simulink model "building_PHPP_v1"  (R2018b)
settings: Solver=ode23s  StartTime=-building.preruntime+8760*3600  StopTime=building.runtime+8760*3600  EnableMultiTasking=on
StartFcn:
  | tic
StopFcn:
  | toc
values from neighbouring files (symbols this model uses):
  A = 7*10*2    (= 140)    [theta_ground_v1.m]    (also in xlswrite1.m = num2cell(data))
  B = A/(0.5 * P)    (= 8.23529411765)    [theta_ground_v1.m]
  building = obj    [BUILDING.m]    (also in create_building_automatic.m = building.save(); ini_building_automatic.m = building.add_variant_hvac(building.variant_hvac, hvac); load_building_automatic.m = building.save())
  C = zeros(1,length(d)+1)    [CONSTRUCTION.m]    (also in DOOR.m = [0 0 0]; WALL.m = [0 0 0]; WINDOW.m = [0 0 0])
  cp = str2num(value)    [CONSTRUCTION.m]
  p = [timevec_weather weather(:,12)]    [BOUNDARY.m]    (also in WEATHER.m = 0; init_carnotUIBK.m = cell2mat(carnotUIBKpaths(i,2)))
  rho = str2num(value)    [CONSTRUCTION.m]    (also in theta_ground_v1.m = 2000)
undefined symbols (not defined in the file or in its folder): Dd, Dreifach, get_building, Qdot_C, Qdot_C_energy, Qdot_H, Qdot_H_energy, Qdot_I_electricity, Qdot_I_electricity_energy, Qdot_I_light, Qdot_I_light_energy, Qdot_I_person, Qdot_I_person_energy, Qdot_S, Qdot_S_energy, Qdot_T_ground, Qdot_T_ground_energy, Qdot_T_neighbour, Qdot_T_neighbour_energy, Qdot_T_opaque, Qdot_T_opaque_energy, Qdot_T_window, Qdot_T_window_energy, Qdot_V_infiltration, Qdot_V_infiltration_energy, Qdot_V_mech, Qdot_V_mech_energy, Qdot_V_window, Qdot_V_window_energy, Tc, Tr, Ts, Wärmeschutzglas, x_CO2, x_H2O, x_VOC
libraries: carnotUIBK x1874, carnot x5, simulink x3
(part 21 of 34)

== system building_PHPP_v1/BUILDING/INTERSECTION_5_8/wall_1 ==
  AIB1 : Inport
  AIB2 : Inport  Port=2
  Qdot_sol1 : Inport  Port=3
  Qdot_sol2 : Inport  Port=4
  EMPTY : carnotUIBK/wall_intersection/EMPTY  VariantControl=(default)
  R-C model : carnotUIBK/wall_intersection/R-C model  VariantControl=V_i_5_8_w1_m1  t0=z.t_ini  d=fliplr(const.parameter.xmesh_beu)  cond=fliplr(const.parameter.lambda)  cwall=fliplr(const.parameter.cp)  rho=fliplr(const.parameter.rho)  reflectground=0.2  abs_emiss=[const.absorption_2 const.emission_2 const.emission_1]  tau=const.parameter.tau  dactive=const.parameter.d_active
      link override alpha_i1/alpha_i_down: VariantControl=V_i_5_8_w1_hti2
      link override alpha_i1/alpha_i_horizontal: VariantControl=V_i_5_8_w1_hti0
      link override alpha_i1/alpha_i_up: VariantControl=V_i_5_8_w1_hti1
      link override alpha_i2/alpha_i_down: VariantControl=V_i_5_8_w1_hti2
      link override alpha_i2/alpha_i_horizontal: VariantControl=V_i_5_8_w1_hti0
      link override alpha_i2/alpha_i_up: VariantControl=V_i_5_8_w1_hti1
  UA : carnotUIBK/wall_intersection/UA  VariantControl=V_i_5_8_w1_m0  U=const.parameter.U
      link override Rsi/down: VariantControl=V_i_5_8_w1_hti2
      link override Rsi/horizontal: VariantControl=V_i_5_8_w1_hti0
      link override Rsi/up: VariantControl=V_i_5_8_w1_hti1
  hygrothermal model : carnotUIBK/wall_intersection/hygrothermal model  VariantControl=V_i_5_8_w1_m2  t0=z.t_ini  reflectground=0.2  abs_emiss=[const.absorption_2 const.emission_2 const.emission_1]  xmesh=const.parameter.xmesh_hygro  X=const.parameter.X  d=const.parameter.d  lambda=const.parameter.lambda_hygro  rho=const.parameter.rho_hygro  cp=const.parameter.cp_hygro  mu=const.parameter.mu  ufs=const.parameter.ufs  FSF_u=const.parameter.FSF_u  FSF_phi=const.parameter.FSF_phi  FSF_dudphi=const.parameter.FSF_dudphi  FSF_k=const.parameter.FSF_k  K_kleff=const.parameter.K_kleff  K_u=const.parameter.K_u  K_kl=const.parameter.K_kl  FSF_length=const.parameter.FSF_length  K_length=const.parameter.K_length  T_ini=const.parameter.T_ini_hygro  Phi_ini=const.parameter.Phi_ini_hygro  T_source=const.parameter.T_source  Phi_source=const.parameter.Phi_source  Tdactive=const.parameter.T_dactive  Phidactive=const.parameter.Phi_dactive
      link override alpha_i1/alpha_i_down: VariantControl=V_i_5_8_w1_hti2
      link override alpha_i1/alpha_i_horizontal: VariantControl=V_i_5_8_w1_hti0
      link override alpha_i1/alpha_i_up: VariantControl=V_i_5_8_w1_hti1
      link override alpha_i2/alpha_i_down: VariantControl=V_i_5_8_w1_hti2
      link override alpha_i2/alpha_i_horizontal: VariantControl=V_i_5_8_w1_hti0
      link override alpha_i2/alpha_i_up: VariantControl=V_i_5_8_w1_hti1
  "[S1]" : Outport
  "[S2]" : Outport  Port=2

== system building_PHPP_v1/BUILDING/INTERSECTION_5_8/wall_2 ==
  AIB1 : Inport
  AIB2 : Inport  Port=2
  Qdot_sol1 : Inport  Port=3
  Qdot_sol2 : Inport  Port=4
  EMPTY : carnotUIBK/wall_intersection/EMPTY  VariantControl=(default)
  R-C model : carnotUIBK/wall_intersection/R-C model  VariantControl=V_i_5_8_w2_m1  t0=z.t_ini  d=fliplr(const.parameter.xmesh_beu)  cond=fliplr(const.parameter.lambda)  cwall=fliplr(const.parameter.cp)  rho=fliplr(const.parameter.rho)  reflectground=0.2  abs_emiss=[const.absorption_2 const.emission_2 const.emission_1]  tau=const.parameter.tau  dactive=const.parameter.d_active
      link override alpha_i1/alpha_i_down: VariantControl=V_i_5_8_w2_hti2
      link override alpha_i1/alpha_i_horizontal: VariantControl=V_i_5_8_w2_hti0
      link override alpha_i1/alpha_i_up: VariantControl=V_i_5_8_w2_hti1
      link override alpha_i2/alpha_i_down: VariantControl=V_i_5_8_w2_hti2
      link override alpha_i2/alpha_i_horizontal: VariantControl=V_i_5_8_w2_hti0
      link override alpha_i2/alpha_i_up: VariantControl=V_i_5_8_w2_hti1
  UA : carnotUIBK/wall_intersection/UA  VariantControl=V_i_5_8_w2_m0  U=const.parameter.U
      link override Rsi/down: VariantControl=V_i_5_8_w2_hti2
      link override Rsi/horizontal: VariantControl=V_i_5_8_w2_hti0
      link override Rsi/up: VariantControl=V_i_5_8_w2_hti1
  hygrothermal model : carnotUIBK/wall_intersection/hygrothermal model  VariantControl=V_i_5_8_w2_m2  t0=z.t_ini  reflectground=0.2  abs_emiss=[const.absorption_2 const.emission_2 const.emission_1]  xmesh=const.parameter.xmesh_hygro  X=const.parameter.X  d=const.parameter.d  lambda=const.parameter.lambda_hygro  rho=const.parameter.rho_hygro  cp=const.parameter.cp_hygro  mu=const.parameter.mu  ufs=const.parameter.ufs  FSF_u=const.parameter.FSF_u  FSF_phi=const.parameter.FSF_phi  FSF_dudphi=const.parameter.FSF_dudphi  FSF_k=const.parameter.FSF_k  K_kleff=const.parameter.K_kleff  K_u=const.parameter.K_u  K_kl=const.parameter.K_kl  FSF_length=const.parameter.FSF_length  K_length=const.parameter.K_length  T_ini=const.parameter.T_ini_hygro  Phi_ini=const.parameter.Phi_ini_hygro  T_source=const.parameter.T_source  Phi_source=const.parameter.Phi_source  Tdactive=const.parameter.T_dactive  Phidactive=const.parameter.Phi_dactive
      link override alpha_i1/alpha_i_down: VariantControl=V_i_5_8_w2_hti2
      link override alpha_i1/alpha_i_horizontal: VariantControl=V_i_5_8_w2_hti0
      link override alpha_i1/alpha_i_up: VariantControl=V_i_5_8_w2_hti1
      link override alpha_i2/alpha_i_down: VariantControl=V_i_5_8_w2_hti2
      link override alpha_i2/alpha_i_horizontal: VariantControl=V_i_5_8_w2_hti0
      link override alpha_i2/alpha_i_up: VariantControl=V_i_5_8_w2_hti1
  "[S1]" : Outport
  "[S2]" : Outport  Port=2

== system building_PHPP_v1/BUILDING/INTERSECTION_5_8/wall_3 ==
  AIB1 : Inport
  AIB2 : Inport  Port=2
  Qdot_sol1 : Inport  Port=3
  Qdot_sol2 : Inport  Port=4
  EMPTY : carnotUIBK/wall_intersection/EMPTY  VariantControl=(default)
  R-C model : carnotUIBK/wall_intersection/R-C model  VariantControl=V_i_5_8_w3_m1  t0=z.t_ini  d=fliplr(const.parameter.xmesh_beu)  cond=fliplr(const.parameter.lambda)  cwall=fliplr(const.parameter.cp)  rho=fliplr(const.parameter.rho)  reflectground=0.2  abs_emiss=[const.absorption_2 const.emission_2 const.emission_1]  tau=const.parameter.tau  dactive=const.parameter.d_active
      link override alpha_i1/alpha_i_down: VariantControl=V_i_5_8_w3_hti2
      link override alpha_i1/alpha_i_horizontal: VariantControl=V_i_5_8_w3_hti0
      link override alpha_i1/alpha_i_up: VariantControl=V_i_5_8_w3_hti1
      link override alpha_i2/alpha_i_down: VariantControl=V_i_5_8_w3_hti2
      link override alpha_i2/alpha_i_horizontal: VariantControl=V_i_5_8_w3_hti0
      link override alpha_i2/alpha_i_up: VariantControl=V_i_5_8_w3_hti1
  UA : carnotUIBK/wall_intersection/UA  VariantControl=V_i_5_8_w3_m0  U=const.parameter.U
      link override Rsi/down: VariantControl=V_i_5_8_w3_hti2
      link override Rsi/horizontal: VariantControl=V_i_5_8_w3_hti0
      link override Rsi/up: VariantControl=V_i_5_8_w3_hti1
  hygrothermal model : carnotUIBK/wall_intersection/hygrothermal model  VariantControl=V_i_5_8_w3_m2  t0=z.t_ini  reflectground=0.2  abs_emiss=[const.absorption_2 const.emission_2 const.emission_1]  xmesh=const.parameter.xmesh_hygro  X=const.parameter.X  d=const.parameter.d  lambda=const.parameter.lambda_hygro  rho=const.parameter.rho_hygro  cp=const.parameter.cp_hygro  mu=const.parameter.mu  ufs=const.parameter.ufs  FSF_u=const.parameter.FSF_u  FSF_phi=const.parameter.FSF_phi  FSF_dudphi=const.parameter.FSF_dudphi  FSF_k=const.parameter.FSF_k  K_kleff=const.parameter.K_kleff  K_u=const.parameter.K_u  K_kl=const.parameter.K_kl  FSF_length=const.parameter.FSF_length  K_length=const.parameter.K_length  T_ini=const.parameter.T_ini_hygro  Phi_ini=const.parameter.Phi_ini_hygro  T_source=const.parameter.T_source  Phi_source=const.parameter.Phi_source  Tdactive=const.parameter.T_dactive  Phidactive=const.parameter.Phi_dactive
      link override alpha_i1/alpha_i_down: VariantControl=V_i_5_8_w3_hti2
      link override alpha_i1/alpha_i_horizontal: VariantControl=V_i_5_8_w3_hti0
      link override alpha_i1/alpha_i_up: VariantControl=V_i_5_8_w3_hti1
      link override alpha_i2/alpha_i_down: VariantControl=V_i_5_8_w3_hti2
      link override alpha_i2/alpha_i_horizontal: VariantControl=V_i_5_8_w3_hti0
      link override alpha_i2/alpha_i_up: VariantControl=V_i_5_8_w3_hti1
  "[S1]" : Outport
  "[S2]" : Outport  Port=2

== system building_PHPP_v1/BUILDING/INTERSECTION_5_9/airexchange_1 ==
  AIB1 : Inport
  AIB2 : Inport  Port=2
  control : Inport  Port=3
  EMPTY : carnotUIBK/airexchange_intersection/EMPTY  VariantControl=(default)
  airexchange_empiric : carnotUIBK/airexchange_intersection/airexchange_empiric  VariantControl=V_i_5_9_inf1_m0
  airexchange_powerlaw : carnotUIBK/airexchange_intersection/airexchange_powerlaw  VariantControl=V_i_5_9_inf1_m1
  "[S1]" : Outport
  "[S2]" : Outport  Port=2

== system building_PHPP_v1/BUILDING/INTERSECTION_5_9/airexchange_2 ==
  AIB1 : Inport
  AIB2 : Inport  Port=2
  control : Inport  Port=3
  EMPTY : carnotUIBK/airexchange_intersection/EMPTY  VariantControl=(default)
  airexchange_empiric : carnotUIBK/airexchange_intersection/airexchange_empiric  VariantControl=V_i_5_9_inf2_m0
  airexchange_powerlaw : carnotUIBK/airexchange_intersection/airexchange_powerlaw  VariantControl=V_i_5_9_inf2_m1
  "[S1]" : Outport
  "[S2]" : Outport  Port=2

== system building_PHPP_v1/BUILDING/INTERSECTION_5_9/airexchange_3 ==
  AIB1 : Inport
  AIB2 : Inport  Port=2
  control : Inport  Port=3
  EMPTY : carnotUIBK/airexchange_intersection/EMPTY  VariantControl=(default)
  airexchange_empiric : carnotUIBK/airexchange_intersection/airexchange_empiric  VariantControl=V_i_5_9_inf3_m0
  airexchange_powerlaw : carnotUIBK/airexchange_intersection/airexchange_powerlaw  VariantControl=V_i_5_9_inf3_m1
  "[S1]" : Outport
  "[S2]" : Outport  Port=2

== system building_PHPP_v1/BUILDING/INTERSECTION_5_9/wall_1 ==
  AIB1 : Inport
  AIB2 : Inport  Port=2
  Qdot_sol1 : Inport  Port=3
  Qdot_sol2 : Inport  Port=4
  EMPTY : carnotUIBK/wall_intersection/EMPTY  VariantControl=(default)
  R-C model : carnotUIBK/wall_intersection/R-C model  VariantControl=V_i_5_9_w1_m1  t0=z.t_ini  d=fliplr(const.parameter.xmesh_beu)  cond=fliplr(const.parameter.lambda)  cwall=fliplr(const.parameter.cp)  rho=fliplr(const.parameter.rho)  reflectground=0.2  abs_emiss=[const.absorption_2 const.emission_2 const.emission_1]  tau=const.parameter.tau  dactive=const.parameter.d_active
      link override alpha_i1/alpha_i_down: VariantControl=V_i_5_9_w1_hti2
      link override alpha_i1/alpha_i_horizontal: VariantControl=V_i_5_9_w1_hti0
      link override alpha_i1/alpha_i_up: VariantControl=V_i_5_9_w1_hti1
      link override alpha_i2/alpha_i_down: VariantControl=V_i_5_9_w1_hti2
      link override alpha_i2/alpha_i_horizontal: VariantControl=V_i_5_9_w1_hti0
      link override alpha_i2/alpha_i_up: VariantControl=V_i_5_9_w1_hti1
  UA : carnotUIBK/wall_intersection/UA  VariantControl=V_i_5_9_w1_m0  U=const.parameter.U
      link override Rsi/down: VariantControl=V_i_5_9_w1_hti2
      link override Rsi/horizontal: VariantControl=V_i_5_9_w1_hti0
      link override Rsi/up: VariantControl=V_i_5_9_w1_hti1
  hygrothermal model : carnotUIBK/wall_intersection/hygrothermal model  VariantControl=V_i_5_9_w1_m2  t0=z.t_ini  reflectground=0.2  abs_emiss=[const.absorption_2 const.emission_2 const.emission_1]  xmesh=const.parameter.xmesh_hygro  X=const.parameter.X  d=const.parameter.d  lambda=const.parameter.lambda_hygro  rho=const.parameter.rho_hygro  cp=const.parameter.cp_hygro  mu=const.parameter.mu  ufs=const.parameter.ufs  FSF_u=const.parameter.FSF_u  FSF_phi=const.parameter.FSF_phi  FSF_dudphi=const.parameter.FSF_dudphi  FSF_k=const.parameter.FSF_k  K_kleff=const.parameter.K_kleff  K_u=const.parameter.K_u  K_kl=const.parameter.K_kl  FSF_length=const.parameter.FSF_length  K_length=const.parameter.K_length  T_ini=const.parameter.T_ini_hygro  Phi_ini=const.parameter.Phi_ini_hygro  T_source=const.parameter.T_source  Phi_source=const.parameter.Phi_source  Tdactive=const.parameter.T_dactive  Phidactive=const.parameter.Phi_dactive
      link override alpha_i1/alpha_i_down: VariantControl=V_i_5_9_w1_hti2
      link override alpha_i1/alpha_i_horizontal: VariantControl=V_i_5_9_w1_hti0
      link override alpha_i1/alpha_i_up: VariantControl=V_i_5_9_w1_hti1
      link override alpha_i2/alpha_i_down: VariantControl=V_i_5_9_w1_hti2
      link override alpha_i2/alpha_i_horizontal: VariantControl=V_i_5_9_w1_hti0
      link override alpha_i2/alpha_i_up: VariantControl=V_i_5_9_w1_hti1
  "[S1]" : Outport
  "[S2]" : Outport  Port=2

== system building_PHPP_v1/BUILDING/INTERSECTION_5_9/wall_2 ==
  AIB1 : Inport
  AIB2 : Inport  Port=2
  Qdot_sol1 : Inport  Port=3
  Qdot_sol2 : Inport  Port=4
  EMPTY : carnotUIBK/wall_intersection/EMPTY  VariantControl=(default)
  R-C model : carnotUIBK/wall_intersection/R-C model  VariantControl=V_i_5_9_w2_m1  t0=z.t_ini  d=fliplr(const.parameter.xmesh_beu)  cond=fliplr(const.parameter.lambda)  cwall=fliplr(const.parameter.cp)  rho=fliplr(const.parameter.rho)  reflectground=0.2  abs_emiss=[const.absorption_2 const.emission_2 const.emission_1]  tau=const.parameter.tau  dactive=const.parameter.d_active
      link override alpha_i1/alpha_i_down: VariantControl=V_i_5_9_w2_hti2
      link override alpha_i1/alpha_i_horizontal: VariantControl=V_i_5_9_w2_hti0
      link override alpha_i1/alpha_i_up: VariantControl=V_i_5_9_w2_hti1
      link override alpha_i2/alpha_i_down: VariantControl=V_i_5_9_w2_hti2
      link override alpha_i2/alpha_i_horizontal: VariantControl=V_i_5_9_w2_hti0
      link override alpha_i2/alpha_i_up: VariantControl=V_i_5_9_w2_hti1
  UA : carnotUIBK/wall_intersection/UA  VariantControl=V_i_5_9_w2_m0  U=const.parameter.U
      link override Rsi/down: VariantControl=V_i_5_9_w2_hti2
      link override Rsi/horizontal: VariantControl=V_i_5_9_w2_hti0
      link override Rsi/up: VariantControl=V_i_5_9_w2_hti1
  hygrothermal model : carnotUIBK/wall_intersection/hygrothermal model  VariantControl=V_i_5_9_w2_m2  t0=z.t_ini  reflectground=0.2  abs_emiss=[const.absorption_2 const.emission_2 const.emission_1]  xmesh=const.parameter.xmesh_hygro  X=const.parameter.X  d=const.parameter.d  lambda=const.parameter.lambda_hygro  rho=const.parameter.rho_hygro  cp=const.parameter.cp_hygro  mu=const.parameter.mu  ufs=const.parameter.ufs  FSF_u=const.parameter.FSF_u  FSF_phi=const.parameter.FSF_phi  FSF_dudphi=const.parameter.FSF_dudphi  FSF_k=const.parameter.FSF_k  K_kleff=const.parameter.K_kleff  K_u=const.parameter.K_u  K_kl=const.parameter.K_kl  FSF_length=const.parameter.FSF_length  K_length=const.parameter.K_length  T_ini=const.parameter.T_ini_hygro  Phi_ini=const.parameter.Phi_ini_hygro  T_source=const.parameter.T_source  Phi_source=const.parameter.Phi_source  Tdactive=const.parameter.T_dactive  Phidactive=const.parameter.Phi_dactive
      link override alpha_i1/alpha_i_down: VariantControl=V_i_5_9_w2_hti2
      link override alpha_i1/alpha_i_horizontal: VariantControl=V_i_5_9_w2_hti0
      link override alpha_i1/alpha_i_up: VariantControl=V_i_5_9_w2_hti1
      link override alpha_i2/alpha_i_down: VariantControl=V_i_5_9_w2_hti2
      link override alpha_i2/alpha_i_horizontal: VariantControl=V_i_5_9_w2_hti0
      link override alpha_i2/alpha_i_up: VariantControl=V_i_5_9_w2_hti1
  "[S1]" : Outport
  "[S2]" : Outport  Port=2

== system building_PHPP_v1/BUILDING/INTERSECTION_5_9/wall_3 ==
  AIB1 : Inport
  AIB2 : Inport  Port=2
  Qdot_sol1 : Inport  Port=3
  Qdot_sol2 : Inport  Port=4
  EMPTY : carnotUIBK/wall_intersection/EMPTY  VariantControl=(default)
  R-C model : carnotUIBK/wall_intersection/R-C model  VariantControl=V_i_5_9_w3_m1  t0=z.t_ini  d=fliplr(const.parameter.xmesh_beu)  cond=fliplr(const.parameter.lambda)  cwall=fliplr(const.parameter.cp)  rho=fliplr(const.parameter.rho)  reflectground=0.2  abs_emiss=[const.absorption_2 const.emission_2 const.emission_1]  tau=const.parameter.tau  dactive=const.parameter.d_active
      link override alpha_i1/alpha_i_down: VariantControl=V_i_5_9_w3_hti2
      link override alpha_i1/alpha_i_horizontal: VariantControl=V_i_5_9_w3_hti0
      link override alpha_i1/alpha_i_up: VariantControl=V_i_5_9_w3_hti1
      link override alpha_i2/alpha_i_down: VariantControl=V_i_5_9_w3_hti2
      link override alpha_i2/alpha_i_horizontal: VariantControl=V_i_5_9_w3_hti0
      link override alpha_i2/alpha_i_up: VariantControl=V_i_5_9_w3_hti1
  UA : carnotUIBK/wall_intersection/UA  VariantControl=V_i_5_9_w3_m0  U=const.parameter.U
      link override Rsi/down: VariantControl=V_i_5_9_w3_hti2
      link override Rsi/horizontal: VariantControl=V_i_5_9_w3_hti0
      link override Rsi/up: VariantControl=V_i_5_9_w3_hti1
  hygrothermal model : carnotUIBK/wall_intersection/hygrothermal model  VariantControl=V_i_5_9_w3_m2  t0=z.t_ini  reflectground=0.2  abs_emiss=[const.absorption_2 const.emission_2 const.emission_1]  xmesh=const.parameter.xmesh_hygro  X=const.parameter.X  d=const.parameter.d  lambda=const.parameter.lambda_hygro  rho=const.parameter.rho_hygro  cp=const.parameter.cp_hygro  mu=const.parameter.mu  ufs=const.parameter.ufs  FSF_u=const.parameter.FSF_u  FSF_phi=const.parameter.FSF_phi  FSF_dudphi=const.parameter.FSF_dudphi  FSF_k=const.parameter.FSF_k  K_kleff=const.parameter.K_kleff  K_u=const.parameter.K_u  K_kl=const.parameter.K_kl  FSF_length=const.parameter.FSF_length  K_length=const.parameter.K_length  T_ini=const.parameter.T_ini_hygro  Phi_ini=const.parameter.Phi_ini_hygro  T_source=const.parameter.T_source  Phi_source=const.parameter.Phi_source  Tdactive=const.parameter.T_dactive  Phidactive=const.parameter.Phi_dactive
      link override alpha_i1/alpha_i_down: VariantControl=V_i_5_9_w3_hti2
      link override alpha_i1/alpha_i_horizontal: VariantControl=V_i_5_9_w3_hti0
      link override alpha_i1/alpha_i_up: VariantControl=V_i_5_9_w3_hti1
      link override alpha_i2/alpha_i_down: VariantControl=V_i_5_9_w3_hti2
      link override alpha_i2/alpha_i_horizontal: VariantControl=V_i_5_9_w3_hti0
      link override alpha_i2/alpha_i_up: VariantControl=V_i_5_9_w3_hti1
  "[S1]" : Outport
  "[S2]" : Outport  Port=2

== system building_PHPP_v1/BUILDING/INTERSECTION_6_10/airexchange_1 ==
  AIB1 : Inport
  AIB2 : Inport  Port=2
  control : Inport  Port=3
  EMPTY : carnotUIBK/airexchange_intersection/EMPTY  VariantControl=(default)
  airexchange_empiric : carnotUIBK/airexchange_intersection/airexchange_empiric  VariantControl=V_i_6_10_inf1_m0
  airexchange_powerlaw : carnotUIBK/airexchange_intersection/airexchange_powerlaw  VariantControl=V_i_6_10_inf1_m1
  "[S1]" : Outport
  "[S2]" : Outport  Port=2

== system building_PHPP_v1/BUILDING/INTERSECTION_6_10/airexchange_2 ==
  AIB1 : Inport
  AIB2 : Inport  Port=2
  control : Inport  Port=3
  EMPTY : carnotUIBK/airexchange_intersection/EMPTY  VariantControl=(default)
  airexchange_empiric : carnotUIBK/airexchange_intersection/airexchange_empiric  VariantControl=V_i_6_10_inf2_m0
  airexchange_powerlaw : carnotUIBK/airexchange_intersection/airexchange_powerlaw  VariantControl=V_i_6_10_inf2_m1
  "[S1]" : Outport
  "[S2]" : Outport  Port=2

== system building_PHPP_v1/BUILDING/INTERSECTION_6_10/airexchange_3 ==
  AIB1 : Inport
  AIB2 : Inport  Port=2
  control : Inport  Port=3
  EMPTY : carnotUIBK/airexchange_intersection/EMPTY  VariantControl=(default)
  airexchange_empiric : carnotUIBK/airexchange_intersection/airexchange_empiric  VariantControl=V_i_6_10_inf3_m0
  airexchange_powerlaw : carnotUIBK/airexchange_intersection/airexchange_powerlaw  VariantControl=V_i_6_10_inf3_m1
  "[S1]" : Outport
  "[S2]" : Outport  Port=2

== system building_PHPP_v1/BUILDING/INTERSECTION_6_10/wall_1 ==
  AIB1 : Inport
  AIB2 : Inport  Port=2
  Qdot_sol1 : Inport  Port=3
  Qdot_sol2 : Inport  Port=4
  EMPTY : carnotUIBK/wall_intersection/EMPTY  VariantControl=(default)
  R-C model : carnotUIBK/wall_intersection/R-C model  VariantControl=V_i_6_10_w1_m1  t0=z.t_ini  d=fliplr(const.parameter.xmesh_beu)  cond=fliplr(const.parameter.lambda)  cwall=fliplr(const.parameter.cp)  rho=fliplr(const.parameter.rho)  reflectground=0.2  abs_emiss=[const.absorption_2 const.emission_2 const.emission_1]  tau=const.parameter.tau  dactive=const.parameter.d_active
      link override alpha_i1/alpha_i_down: VariantControl=V_i_6_10_w1_hti2
      link override alpha_i1/alpha_i_horizontal: VariantControl=V_i_6_10_w1_hti0
      link override alpha_i1/alpha_i_up: VariantControl=V_i_6_10_w1_hti1
      link override alpha_i2/alpha_i_down: VariantControl=V_i_6_10_w1_hti2
      link override alpha_i2/alpha_i_horizontal: VariantControl=V_i_6_10_w1_hti0
      link override alpha_i2/alpha_i_up: VariantControl=V_i_6_10_w1_hti1
  UA : carnotUIBK/wall_intersection/UA  VariantControl=V_i_6_10_w1_m0  U=const.parameter.U
      link override Rsi/down: VariantControl=V_i_6_10_w1_hti2
      link override Rsi/horizontal: VariantControl=V_i_6_10_w1_hti0
      link override Rsi/up: VariantControl=V_i_6_10_w1_hti1
  hygrothermal model : carnotUIBK/wall_intersection/hygrothermal model  VariantControl=V_i_6_10_w1_m2  t0=z.t_ini  reflectground=0.2  abs_emiss=[const.absorption_2 const.emission_2 const.emission_1]  xmesh=const.parameter.xmesh_hygro  X=const.parameter.X  d=const.parameter.d  lambda=const.parameter.lambda_hygro  rho=const.parameter.rho_hygro  cp=const.parameter.cp_hygro  mu=const.parameter.mu  ufs=const.parameter.ufs  FSF_u=const.parameter.FSF_u  FSF_phi=const.parameter.FSF_phi  FSF_dudphi=const.parameter.FSF_dudphi  FSF_k=const.parameter.FSF_k  K_kleff=const.parameter.K_kleff  K_u=const.parameter.K_u  K_kl=const.parameter.K_kl  FSF_length=const.parameter.FSF_length  K_length=const.parameter.K_length  T_ini=const.parameter.T_ini_hygro  Phi_ini=const.parameter.Phi_ini_hygro  T_source=const.parameter.T_source  Phi_source=const.parameter.Phi_source  Tdactive=const.parameter.T_dactive  Phidactive=const.parameter.Phi_dactive
      link override alpha_i1/alpha_i_down: VariantControl=V_i_6_10_w1_hti2
      link override alpha_i1/alpha_i_horizontal: VariantControl=V_i_6_10_w1_hti0
      link override alpha_i1/alpha_i_up: VariantControl=V_i_6_10_w1_hti1
      link override alpha_i2/alpha_i_down: VariantControl=V_i_6_10_w1_hti2
      link override alpha_i2/alpha_i_horizontal: VariantControl=V_i_6_10_w1_hti0
      link override alpha_i2/alpha_i_up: VariantControl=V_i_6_10_w1_hti1
  "[S1]" : Outport
  "[S2]" : Outport  Port=2

== system building_PHPP_v1/BUILDING/INTERSECTION_6_10/wall_2 ==
  AIB1 : Inport
  AIB2 : Inport  Port=2
  Qdot_sol1 : Inport  Port=3
  Qdot_sol2 : Inport  Port=4
  EMPTY : carnotUIBK/wall_intersection/EMPTY  VariantControl=(default)
  R-C model : carnotUIBK/wall_intersection/R-C model  VariantControl=V_i_6_10_w2_m1  t0=z.t_ini  d=fliplr(const.parameter.xmesh_beu)  cond=fliplr(const.parameter.lambda)  cwall=fliplr(const.parameter.cp)  rho=fliplr(const.parameter.rho)  reflectground=0.2  abs_emiss=[const.absorption_2 const.emission_2 const.emission_1]  tau=const.parameter.tau  dactive=const.parameter.d_active
      link override alpha_i1/alpha_i_down: VariantControl=V_i_6_10_w2_hti2
      link override alpha_i1/alpha_i_horizontal: VariantControl=V_i_6_10_w2_hti0
      link override alpha_i1/alpha_i_up: VariantControl=V_i_6_10_w2_hti1
      link override alpha_i2/alpha_i_down: VariantControl=V_i_6_10_w2_hti2
      link override alpha_i2/alpha_i_horizontal: VariantControl=V_i_6_10_w2_hti0
      link override alpha_i2/alpha_i_up: VariantControl=V_i_6_10_w2_hti1
  UA : carnotUIBK/wall_intersection/UA  VariantControl=V_i_6_10_w2_m0  U=const.parameter.U
      link override Rsi/down: VariantControl=V_i_6_10_w2_hti2
      link override Rsi/horizontal: VariantControl=V_i_6_10_w2_hti0
      link override Rsi/up: VariantControl=V_i_6_10_w2_hti1
  hygrothermal model : carnotUIBK/wall_intersection/hygrothermal model  VariantControl=V_i_6_10_w2_m2  t0=z.t_ini  reflectground=0.2  abs_emiss=[const.absorption_2 const.emission_2 const.emission_1]  xmesh=const.parameter.xmesh_hygro  X=const.parameter.X  d=const.parameter.d  lambda=const.parameter.lambda_hygro  rho=const.parameter.rho_hygro  cp=const.parameter.cp_hygro  mu=const.parameter.mu  ufs=const.parameter.ufs  FSF_u=const.parameter.FSF_u  FSF_phi=const.parameter.FSF_phi  FSF_dudphi=const.parameter.FSF_dudphi  FSF_k=const.parameter.FSF_k  K_kleff=const.parameter.K_kleff  K_u=const.parameter.K_u  K_kl=const.parameter.K_kl  FSF_length=const.parameter.FSF_length  K_length=const.parameter.K_length  T_ini=const.parameter.T_ini_hygro  Phi_ini=const.parameter.Phi_ini_hygro  T_source=const.parameter.T_source  Phi_source=const.parameter.Phi_source  Tdactive=const.parameter.T_dactive  Phidactive=const.parameter.Phi_dactive
      link override alpha_i1/alpha_i_down: VariantControl=V_i_6_10_w2_hti2
      link override alpha_i1/alpha_i_horizontal: VariantControl=V_i_6_10_w2_hti0
      link override alpha_i1/alpha_i_up: VariantControl=V_i_6_10_w2_hti1
      link override alpha_i2/alpha_i_down: VariantControl=V_i_6_10_w2_hti2
      link override alpha_i2/alpha_i_horizontal: VariantControl=V_i_6_10_w2_hti0
      link override alpha_i2/alpha_i_up: VariantControl=V_i_6_10_w2_hti1
  "[S1]" : Outport
  "[S2]" : Outport  Port=2

== system building_PHPP_v1/BUILDING/INTERSECTION_6_10/wall_3 ==
  AIB1 : Inport
  AIB2 : Inport  Port=2
  Qdot_sol1 : Inport  Port=3
  Qdot_sol2 : Inport  Port=4
  EMPTY : carnotUIBK/wall_intersection/EMPTY  VariantControl=(default)
  R-C model : carnotUIBK/wall_intersection/R-C model  VariantControl=V_i_6_10_w3_m1  t0=z.t_ini  d=fliplr(const.parameter.xmesh_beu)  cond=fliplr(const.parameter.lambda)  cwall=fliplr(const.parameter.cp)  rho=fliplr(const.parameter.rho)  reflectground=0.2  abs_emiss=[const.absorption_2 const.emission_2 const.emission_1]  tau=const.parameter.tau  dactive=const.parameter.d_active
      link override alpha_i1/alpha_i_down: VariantControl=V_i_6_10_w3_hti2
      link override alpha_i1/alpha_i_horizontal: VariantControl=V_i_6_10_w3_hti0
      link override alpha_i1/alpha_i_up: VariantControl=V_i_6_10_w3_hti1
      link override alpha_i2/alpha_i_down: VariantControl=V_i_6_10_w3_hti2
      link override alpha_i2/alpha_i_horizontal: VariantControl=V_i_6_10_w3_hti0
      link override alpha_i2/alpha_i_up: VariantControl=V_i_6_10_w3_hti1
  UA : carnotUIBK/wall_intersection/UA  VariantControl=V_i_6_10_w3_m0  U=const.parameter.U
      link override Rsi/down: VariantControl=V_i_6_10_w3_hti2
      link override Rsi/horizontal: VariantControl=V_i_6_10_w3_hti0
      link override Rsi/up: VariantControl=V_i_6_10_w3_hti1
  hygrothermal model : carnotUIBK/wall_intersection/hygrothermal model  VariantControl=V_i_6_10_w3_m2  t0=z.t_ini  reflectground=0.2  abs_emiss=[const.absorption_2 const.emission_2 const.emission_1]  xmesh=const.parameter.xmesh_hygro  X=const.parameter.X  d=const.parameter.d  lambda=const.parameter.lambda_hygro  rho=const.parameter.rho_hygro  cp=const.parameter.cp_hygro  mu=const.parameter.mu  ufs=const.parameter.ufs  FSF_u=const.parameter.FSF_u  FSF_phi=const.parameter.FSF_phi  FSF_dudphi=const.parameter.FSF_dudphi  FSF_k=const.parameter.FSF_k  K_kleff=const.parameter.K_kleff  K_u=const.parameter.K_u  K_kl=const.parameter.K_kl  FSF_length=const.parameter.FSF_length  K_length=const.parameter.K_length  T_ini=const.parameter.T_ini_hygro  Phi_ini=const.parameter.Phi_ini_hygro  T_source=const.parameter.T_source  Phi_source=const.parameter.Phi_source  Tdactive=const.parameter.T_dactive  Phidactive=const.parameter.Phi_dactive
      link override alpha_i1/alpha_i_down: VariantControl=V_i_6_10_w3_hti2
      link override alpha_i1/alpha_i_horizontal: VariantControl=V_i_6_10_w3_hti0
      link override alpha_i1/alpha_i_up: VariantControl=V_i_6_10_w3_hti1
      link override alpha_i2/alpha_i_down: VariantControl=V_i_6_10_w3_hti2
      link override alpha_i2/alpha_i_horizontal: VariantControl=V_i_6_10_w3_hti0
      link override alpha_i2/alpha_i_up: VariantControl=V_i_6_10_w3_hti1
  "[S1]" : Outport
  "[S2]" : Outport  Port=2

== system building_PHPP_v1/BUILDING/INTERSECTION_6_7/airexchange_1 ==
  AIB1 : Inport
  AIB2 : Inport  Port=2
  control : Inport  Port=3
  EMPTY : carnotUIBK/airexchange_intersection/EMPTY  VariantControl=(default)
  airexchange_empiric : carnotUIBK/airexchange_intersection/airexchange_empiric  VariantControl=V_i_6_7_inf1_m0
  airexchange_powerlaw : carnotUIBK/airexchange_intersection/airexchange_powerlaw  VariantControl=V_i_6_7_inf1_m1
  "[S1]" : Outport
  "[S2]" : Outport  Port=2

== system building_PHPP_v1/BUILDING/INTERSECTION_6_7/airexchange_2 ==
  AIB1 : Inport
  AIB2 : Inport  Port=2
  control : Inport  Port=3
  EMPTY : carnotUIBK/airexchange_intersection/EMPTY  VariantControl=(default)
  airexchange_empiric : carnotUIBK/airexchange_intersection/airexchange_empiric  VariantControl=V_i_6_7_inf2_m0
  airexchange_powerlaw : carnotUIBK/airexchange_intersection/airexchange_powerlaw  VariantControl=V_i_6_7_inf2_m1
  "[S1]" : Outport
  "[S2]" : Outport  Port=2

== system building_PHPP_v1/BUILDING/INTERSECTION_6_7/airexchange_3 ==
  AIB1 : Inport
  AIB2 : Inport  Port=2
  control : Inport  Port=3
  EMPTY : carnotUIBK/airexchange_intersection/EMPTY  VariantControl=(default)
  airexchange_empiric : carnotUIBK/airexchange_intersection/airexchange_empiric  VariantControl=V_i_6_7_inf3_m0
  airexchange_powerlaw : carnotUIBK/airexchange_intersection/airexchange_powerlaw  VariantControl=V_i_6_7_inf3_m1
  "[S1]" : Outport
  "[S2]" : Outport  Port=2

== system building_PHPP_v1/BUILDING/INTERSECTION_6_7/wall_1 ==
  AIB1 : Inport
  AIB2 : Inport  Port=2
  Qdot_sol1 : Inport  Port=3
  Qdot_sol2 : Inport  Port=4
  EMPTY : carnotUIBK/wall_intersection/EMPTY  VariantControl=(default)
  R-C model : carnotUIBK/wall_intersection/R-C model  VariantControl=V_i_6_7_w1_m1  t0=z.t_ini  d=fliplr(const.parameter.xmesh_beu)  cond=fliplr(const.parameter.lambda)  cwall=fliplr(const.parameter.cp)  rho=fliplr(const.parameter.rho)  reflectground=0.2  abs_emiss=[const.absorption_2 const.emission_2 const.emission_1]  tau=const.parameter.tau  dactive=const.parameter.d_active
      link override alpha_i1/alpha_i_down: VariantControl=V_i_6_7_w1_hti2
      link override alpha_i1/alpha_i_horizontal: VariantControl=V_i_6_7_w1_hti0
      link override alpha_i1/alpha_i_up: VariantControl=V_i_6_7_w1_hti1
      link override alpha_i2/alpha_i_down: VariantControl=V_i_6_7_w1_hti2
      link override alpha_i2/alpha_i_horizontal: VariantControl=V_i_6_7_w1_hti0
      link override alpha_i2/alpha_i_up: VariantControl=V_i_6_7_w1_hti1
  UA : carnotUIBK/wall_intersection/UA  VariantControl=V_i_6_7_w1_m0  U=const.parameter.U
      link override Rsi/down: VariantControl=V_i_6_7_w1_hti2
      link override Rsi/horizontal: VariantControl=V_i_6_7_w1_hti0
      link override Rsi/up: VariantControl=V_i_6_7_w1_hti1
  hygrothermal model : carnotUIBK/wall_intersection/hygrothermal model  VariantControl=V_i_6_7_w1_m2  t0=z.t_ini  reflectground=0.2  abs_emiss=[const.absorption_2 const.emission_2 const.emission_1]  xmesh=const.parameter.xmesh_hygro  X=const.parameter.X  d=const.parameter.d  lambda=const.parameter.lambda_hygro  rho=const.parameter.rho_hygro  cp=const.parameter.cp_hygro  mu=const.parameter.mu  ufs=const.parameter.ufs  FSF_u=const.parameter.FSF_u  FSF_phi=const.parameter.FSF_phi  FSF_dudphi=const.parameter.FSF_dudphi  FSF_k=const.parameter.FSF_k  K_kleff=const.parameter.K_kleff  K_u=const.parameter.K_u  K_kl=const.parameter.K_kl  FSF_length=const.parameter.FSF_length  K_length=const.parameter.K_length  T_ini=const.parameter.T_ini_hygro  Phi_ini=const.parameter.Phi_ini_hygro  T_source=const.parameter.T_source  Phi_source=const.parameter.Phi_source  Tdactive=const.parameter.T_dactive  Phidactive=const.parameter.Phi_dactive
      link override alpha_i1/alpha_i_down: VariantControl=V_i_6_7_w1_hti2
      link override alpha_i1/alpha_i_horizontal: VariantControl=V_i_6_7_w1_hti0
      link override alpha_i1/alpha_i_up: VariantControl=V_i_6_7_w1_hti1
      link override alpha_i2/alpha_i_down: VariantControl=V_i_6_7_w1_hti2
      link override alpha_i2/alpha_i_horizontal: VariantControl=V_i_6_7_w1_hti0
      link override alpha_i2/alpha_i_up: VariantControl=V_i_6_7_w1_hti1
  "[S1]" : Outport
  "[S2]" : Outport  Port=2

== system building_PHPP_v1/BUILDING/INTERSECTION_6_7/wall_2 ==
  AIB1 : Inport
  AIB2 : Inport  Port=2
  Qdot_sol1 : Inport  Port=3
  Qdot_sol2 : Inport  Port=4
  EMPTY : carnotUIBK/wall_intersection/EMPTY  VariantControl=(default)
  R-C model : carnotUIBK/wall_intersection/R-C model  VariantControl=V_i_6_7_w2_m1  t0=z.t_ini  d=fliplr(const.parameter.xmesh_beu)  cond=fliplr(const.parameter.lambda)  cwall=fliplr(const.parameter.cp)  rho=fliplr(const.parameter.rho)  reflectground=0.2  abs_emiss=[const.absorption_2 const.emission_2 const.emission_1]  tau=const.parameter.tau  dactive=const.parameter.d_active
      link override alpha_i1/alpha_i_down: VariantControl=V_i_6_7_w2_hti2
      link override alpha_i1/alpha_i_horizontal: VariantControl=V_i_6_7_w2_hti0
      link override alpha_i1/alpha_i_up: VariantControl=V_i_6_7_w2_hti1
      link override alpha_i2/alpha_i_down: VariantControl=V_i_6_7_w2_hti2
      link override alpha_i2/alpha_i_horizontal: VariantControl=V_i_6_7_w2_hti0
      link override alpha_i2/alpha_i_up: VariantControl=V_i_6_7_w2_hti1
  UA : carnotUIBK/wall_intersection/UA  VariantControl=V_i_6_7_w2_m0  U=const.parameter.U
      link override Rsi/down: VariantControl=V_i_6_7_w2_hti2
      link override Rsi/horizontal: VariantControl=V_i_6_7_w2_hti0
      link override Rsi/up: VariantControl=V_i_6_7_w2_hti1
  hygrothermal model : carnotUIBK/wall_intersection/hygrothermal model  VariantControl=V_i_6_7_w2_m2  t0=z.t_ini  reflectground=0.2  abs_emiss=[const.absorption_2 const.emission_2 const.emission_1]  xmesh=const.parameter.xmesh_hygro  X=const.parameter.X  d=const.parameter.d  lambda=const.parameter.lambda_hygro  rho=const.parameter.rho_hygro  cp=const.parameter.cp_hygro  mu=const.parameter.mu  ufs=const.parameter.ufs  FSF_u=const.parameter.FSF_u  FSF_phi=const.parameter.FSF_phi  FSF_dudphi=const.parameter.FSF_dudphi  FSF_k=const.parameter.FSF_k  K_kleff=const.parameter.K_kleff  K_u=const.parameter.K_u  K_kl=const.parameter.K_kl  FSF_length=const.parameter.FSF_length  K_length=const.parameter.K_length  T_ini=const.parameter.T_ini_hygro  Phi_ini=const.parameter.Phi_ini_hygro  T_source=const.parameter.T_source  Phi_source=const.parameter.Phi_source  Tdactive=const.parameter.T_dactive  Phidactive=const.parameter.Phi_dactive
      link override alpha_i1/alpha_i_down: VariantControl=V_i_6_7_w2_hti2
      link override alpha_i1/alpha_i_horizontal: VariantControl=V_i_6_7_w2_hti0
      link override alpha_i1/alpha_i_up: VariantControl=V_i_6_7_w2_hti1
      link override alpha_i2/alpha_i_down: VariantControl=V_i_6_7_w2_hti2
      link override alpha_i2/alpha_i_horizontal: VariantControl=V_i_6_7_w2_hti0
      link override alpha_i2/alpha_i_up: VariantControl=V_i_6_7_w2_hti1
  "[S1]" : Outport
  "[S2]" : Outport  Port=2

== system building_PHPP_v1/BUILDING/INTERSECTION_6_7/wall_3 ==
  AIB1 : Inport
  AIB2 : Inport  Port=2
  Qdot_sol1 : Inport  Port=3
  Qdot_sol2 : Inport  Port=4
  EMPTY : carnotUIBK/wall_intersection/EMPTY  VariantControl=(default)
  R-C model : carnotUIBK/wall_intersection/R-C model  VariantControl=V_i_6_7_w3_m1  t0=z.t_ini  d=fliplr(const.parameter.xmesh_beu)  cond=fliplr(const.parameter.lambda)  cwall=fliplr(const.parameter.cp)  rho=fliplr(const.parameter.rho)  reflectground=0.2  abs_emiss=[const.absorption_2 const.emission_2 const.emission_1]  tau=const.parameter.tau  dactive=const.parameter.d_active
      link override alpha_i1/alpha_i_down: VariantControl=V_i_6_7_w3_hti2
      link override alpha_i1/alpha_i_horizontal: VariantControl=V_i_6_7_w3_hti0
      link override alpha_i1/alpha_i_up: VariantControl=V_i_6_7_w3_hti1
      link override alpha_i2/alpha_i_down: VariantControl=V_i_6_7_w3_hti2
      link override alpha_i2/alpha_i_horizontal: VariantControl=V_i_6_7_w3_hti0
      link override alpha_i2/alpha_i_up: VariantControl=V_i_6_7_w3_hti1
  UA : carnotUIBK/wall_intersection/UA  VariantControl=V_i_6_7_w3_m0  U=const.parameter.U
      link override Rsi/down: VariantControl=V_i_6_7_w3_hti2
      link override Rsi/horizontal: VariantControl=V_i_6_7_w3_hti0
      link override Rsi/up: VariantControl=V_i_6_7_w3_hti1
  hygrothermal model : carnotUIBK/wall_intersection/hygrothermal model  VariantControl=V_i_6_7_w3_m2  t0=z.t_ini  reflectground=0.2  abs_emiss=[const.absorption_2 const.emission_2 const.emission_1]  xmesh=const.parameter.xmesh_hygro  X=const.parameter.X  d=const.parameter.d  lambda=const.parameter.lambda_hygro  rho=const.parameter.rho_hygro  cp=const.parameter.cp_hygro  mu=const.parameter.mu  ufs=const.parameter.ufs  FSF_u=const.parameter.FSF_u  FSF_phi=const.parameter.FSF_phi  FSF_dudphi=const.parameter.FSF_dudphi  FSF_k=const.parameter.FSF_k  K_kleff=const.parameter.K_kleff  K_u=const.parameter.K_u  K_kl=const.parameter.K_kl  FSF_length=const.parameter.FSF_length  K_length=const.parameter.K_length  T_ini=const.parameter.T_ini_hygro  Phi_ini=const.parameter.Phi_ini_hygro  T_source=const.parameter.T_source  Phi_source=const.parameter.Phi_source  Tdactive=const.parameter.T_dactive  Phidactive=const.parameter.Phi_dactive
      link override alpha_i1/alpha_i_down: VariantControl=V_i_6_7_w3_hti2
      link override alpha_i1/alpha_i_horizontal: VariantControl=V_i_6_7_w3_hti0
      link override alpha_i1/alpha_i_up: VariantControl=V_i_6_7_w3_hti1
      link override alpha_i2/alpha_i_down: VariantControl=V_i_6_7_w3_hti2
      link override alpha_i2/alpha_i_horizontal: VariantControl=V_i_6_7_w3_hti0
      link override alpha_i2/alpha_i_up: VariantControl=V_i_6_7_w3_hti1
  "[S1]" : Outport
  "[S2]" : Outport  Port=2

== system building_PHPP_v1/BUILDING/INTERSECTION_6_8/airexchange_1 ==
  AIB1 : Inport
  AIB2 : Inport  Port=2
  control : Inport  Port=3
  EMPTY : carnotUIBK/airexchange_intersection/EMPTY  VariantControl=(default)
  airexchange_empiric : carnotUIBK/airexchange_intersection/airexchange_empiric  VariantControl=V_i_6_8_inf1_m0
  airexchange_powerlaw : carnotUIBK/airexchange_intersection/airexchange_powerlaw  VariantControl=V_i_6_8_inf1_m1
  "[S1]" : Outport
  "[S2]" : Outport  Port=2

== system building_PHPP_v1/BUILDING/INTERSECTION_6_8/airexchange_2 ==
  AIB1 : Inport
  AIB2 : Inport  Port=2
  control : Inport  Port=3
  EMPTY : carnotUIBK/airexchange_intersection/EMPTY  VariantControl=(default)
  airexchange_empiric : carnotUIBK/airexchange_intersection/airexchange_empiric  VariantControl=V_i_6_8_inf2_m0
  airexchange_powerlaw : carnotUIBK/airexchange_intersection/airexchange_powerlaw  VariantControl=V_i_6_8_inf2_m1
  "[S1]" : Outport
  "[S2]" : Outport  Port=2

== system building_PHPP_v1/BUILDING/INTERSECTION_6_8/airexchange_3 ==
  AIB1 : Inport
  AIB2 : Inport  Port=2
  control : Inport  Port=3
  EMPTY : carnotUIBK/airexchange_intersection/EMPTY  VariantControl=(default)
  airexchange_empiric : carnotUIBK/airexchange_intersection/airexchange_empiric  VariantControl=V_i_6_8_inf3_m0
  airexchange_powerlaw : carnotUIBK/airexchange_intersection/airexchange_powerlaw  VariantControl=V_i_6_8_inf3_m1
  "[S1]" : Outport
  "[S2]" : Outport  Port=2

== system building_PHPP_v1/BUILDING/INTERSECTION_6_8/wall_1 ==
  AIB1 : Inport
  AIB2 : Inport  Port=2
  Qdot_sol1 : Inport  Port=3
  Qdot_sol2 : Inport  Port=4
  EMPTY : carnotUIBK/wall_intersection/EMPTY  VariantControl=(default)
  R-C model : carnotUIBK/wall_intersection/R-C model  VariantControl=V_i_6_8_w1_m1  t0=z.t_ini  d=fliplr(const.parameter.xmesh_beu)  cond=fliplr(const.parameter.lambda)  cwall=fliplr(const.parameter.cp)  rho=fliplr(const.parameter.rho)  reflectground=0.2  abs_emiss=[const.absorption_2 const.emission_2 const.emission_1]  tau=const.parameter.tau  dactive=const.parameter.d_active
      link override alpha_i1/alpha_i_down: VariantControl=V_i_6_8_w1_hti2
      link override alpha_i1/alpha_i_horizontal: VariantControl=V_i_6_8_w1_hti0
      link override alpha_i1/alpha_i_up: VariantControl=V_i_6_8_w1_hti1
      link override alpha_i2/alpha_i_down: VariantControl=V_i_6_8_w1_hti2
      link override alpha_i2/alpha_i_horizontal: VariantControl=V_i_6_8_w1_hti0
      link override alpha_i2/alpha_i_up: VariantControl=V_i_6_8_w1_hti1
  UA : carnotUIBK/wall_intersection/UA  VariantControl=V_i_6_8_w1_m0  U=const.parameter.U
      link override Rsi/down: VariantControl=V_i_6_8_w1_hti2
      link override Rsi/horizontal: VariantControl=V_i_6_8_w1_hti0
      link override Rsi/up: VariantControl=V_i_6_8_w1_hti1
  hygrothermal model : carnotUIBK/wall_intersection/hygrothermal model  VariantControl=V_i_6_8_w1_m2  t0=z.t_ini  reflectground=0.2  abs_emiss=[const.absorption_2 const.emission_2 const.emission_1]  xmesh=const.parameter.xmesh_hygro  X=const.parameter.X  d=const.parameter.d  lambda=const.parameter.lambda_hygro  rho=const.parameter.rho_hygro  cp=const.parameter.cp_hygro  mu=const.parameter.mu  ufs=const.parameter.ufs  FSF_u=const.parameter.FSF_u  FSF_phi=const.parameter.FSF_phi  FSF_dudphi=const.parameter.FSF_dudphi  FSF_k=const.parameter.FSF_k  K_kleff=const.parameter.K_kleff  K_u=const.parameter.K_u  K_kl=const.parameter.K_kl  FSF_length=const.parameter.FSF_length  K_length=const.parameter.K_length  T_ini=const.parameter.T_ini_hygro  Phi_ini=const.parameter.Phi_ini_hygro  T_source=const.parameter.T_source  Phi_source=const.parameter.Phi_source  Tdactive=const.parameter.T_dactive  Phidactive=const.parameter.Phi_dactive
      link override alpha_i1/alpha_i_down: VariantControl=V_i_6_8_w1_hti2
      link override alpha_i1/alpha_i_horizontal: VariantControl=V_i_6_8_w1_hti0
      link override alpha_i1/alpha_i_up: VariantControl=V_i_6_8_w1_hti1
      link override alpha_i2/alpha_i_down: VariantControl=V_i_6_8_w1_hti2
      link override alpha_i2/alpha_i_horizontal: VariantControl=V_i_6_8_w1_hti0
      link override alpha_i2/alpha_i_up: VariantControl=V_i_6_8_w1_hti1
  "[S1]" : Outport
  "[S2]" : Outport  Port=2

== system building_PHPP_v1/BUILDING/INTERSECTION_6_8/wall_2 ==
  AIB1 : Inport
  AIB2 : Inport  Port=2
  Qdot_sol1 : Inport  Port=3
  Qdot_sol2 : Inport  Port=4
  EMPTY : carnotUIBK/wall_intersection/EMPTY  VariantControl=(default)
  R-C model : carnotUIBK/wall_intersection/R-C model  VariantControl=V_i_6_8_w2_m1  t0=z.t_ini  d=fliplr(const.parameter.xmesh_beu)  cond=fliplr(const.parameter.lambda)  cwall=fliplr(const.parameter.cp)  rho=fliplr(const.parameter.rho)  reflectground=0.2  abs_emiss=[const.absorption_2 const.emission_2 const.emission_1]  tau=const.parameter.tau  dactive=const.parameter.d_active
      link override alpha_i1/alpha_i_down: VariantControl=V_i_6_8_w2_hti2
      link override alpha_i1/alpha_i_horizontal: VariantControl=V_i_6_8_w2_hti0
      link override alpha_i1/alpha_i_up: VariantControl=V_i_6_8_w2_hti1
      link override alpha_i2/alpha_i_down: VariantControl=V_i_6_8_w2_hti2
      link override alpha_i2/alpha_i_horizontal: VariantControl=V_i_6_8_w2_hti0
      link override alpha_i2/alpha_i_up: VariantControl=V_i_6_8_w2_hti1
  UA : carnotUIBK/wall_intersection/UA  VariantControl=V_i_6_8_w2_m0  U=const.parameter.U
      link override Rsi/down: VariantControl=V_i_6_8_w2_hti2
      link override Rsi/horizontal: VariantControl=V_i_6_8_w2_hti0
      link override Rsi/up: VariantControl=V_i_6_8_w2_hti1
  hygrothermal model : carnotUIBK/wall_intersection/hygrothermal model  VariantControl=V_i_6_8_w2_m2  t0=z.t_ini  reflectground=0.2  abs_emiss=[const.absorption_2 const.emission_2 const.emission_1]  xmesh=const.parameter.xmesh_hygro  X=const.parameter.X  d=const.parameter.d  lambda=const.parameter.lambda_hygro  rho=const.parameter.rho_hygro  cp=const.parameter.cp_hygro  mu=const.parameter.mu  ufs=const.parameter.ufs  FSF_u=const.parameter.FSF_u  FSF_phi=const.parameter.FSF_phi  FSF_dudphi=const.parameter.FSF_dudphi  FSF_k=const.parameter.FSF_k  K_kleff=const.parameter.K_kleff  K_u=const.parameter.K_u  K_kl=const.parameter.K_kl  FSF_length=const.parameter.FSF_length  K_length=const.parameter.K_length  T_ini=const.parameter.T_ini_hygro  Phi_ini=const.parameter.Phi_ini_hygro  T_source=const.parameter.T_source  Phi_source=const.parameter.Phi_source  Tdactive=const.parameter.T_dactive  Phidactive=const.parameter.Phi_dactive
      link override alpha_i1/alpha_i_down: VariantControl=V_i_6_8_w2_hti2
      link override alpha_i1/alpha_i_horizontal: VariantControl=V_i_6_8_w2_hti0
      link override alpha_i1/alpha_i_up: VariantControl=V_i_6_8_w2_hti1
      link override alpha_i2/alpha_i_down: VariantControl=V_i_6_8_w2_hti2
      link override alpha_i2/alpha_i_horizontal: VariantControl=V_i_6_8_w2_hti0
      link override alpha_i2/alpha_i_up: VariantControl=V_i_6_8_w2_hti1
  "[S1]" : Outport
  "[S2]" : Outport  Port=2

== system building_PHPP_v1/BUILDING/INTERSECTION_6_8/wall_3 ==
  AIB1 : Inport
  AIB2 : Inport  Port=2
  Qdot_sol1 : Inport  Port=3
  Qdot_sol2 : Inport  Port=4
  EMPTY : carnotUIBK/wall_intersection/EMPTY  VariantControl=(default)
  R-C model : carnotUIBK/wall_intersection/R-C model  VariantControl=V_i_6_8_w3_m1  t0=z.t_ini  d=fliplr(const.parameter.xmesh_beu)  cond=fliplr(const.parameter.lambda)  cwall=fliplr(const.parameter.cp)  rho=fliplr(const.parameter.rho)  reflectground=0.2  abs_emiss=[const.absorption_2 const.emission_2 const.emission_1]  tau=const.parameter.tau  dactive=const.parameter.d_active
      link override alpha_i1/alpha_i_down: VariantControl=V_i_6_8_w3_hti2
      link override alpha_i1/alpha_i_horizontal: VariantControl=V_i_6_8_w3_hti0
      link override alpha_i1/alpha_i_up: VariantControl=V_i_6_8_w3_hti1
      link override alpha_i2/alpha_i_down: VariantControl=V_i_6_8_w3_hti2
      link override alpha_i2/alpha_i_horizontal: VariantControl=V_i_6_8_w3_hti0
      link override alpha_i2/alpha_i_up: VariantControl=V_i_6_8_w3_hti1
  UA : carnotUIBK/wall_intersection/UA  VariantControl=V_i_6_8_w3_m0  U=const.parameter.U
      link override Rsi/down: VariantControl=V_i_6_8_w3_hti2
      link override Rsi/horizontal: VariantControl=V_i_6_8_w3_hti0
      link override Rsi/up: VariantControl=V_i_6_8_w3_hti1
  hygrothermal model : carnotUIBK/wall_intersection/hygrothermal model  VariantControl=V_i_6_8_w3_m2  t0=z.t_ini  reflectground=0.2  abs_emiss=[const.absorption_2 const.emission_2 const.emission_1]  xmesh=const.parameter.xmesh_hygro  X=const.parameter.X  d=const.parameter.d  lambda=const.parameter.lambda_hygro  rho=const.parameter.rho_hygro  cp=const.parameter.cp_hygro  mu=const.parameter.mu  ufs=const.parameter.ufs  FSF_u=const.parameter.FSF_u  FSF_phi=const.parameter.FSF_phi  FSF_dudphi=const.parameter.FSF_dudphi  FSF_k=const.parameter.FSF_k  K_kleff=const.parameter.K_kleff  K_u=const.parameter.K_u  K_kl=const.parameter.K_kl  FSF_length=const.parameter.FSF_length  K_length=const.parameter.K_length  T_ini=const.parameter.T_ini_hygro  Phi_ini=const.parameter.Phi_ini_hygro  T_source=const.parameter.T_source  Phi_source=const.parameter.Phi_source  Tdactive=const.parameter.T_dactive  Phidactive=const.parameter.Phi_dactive
      link override alpha_i1/alpha_i_down: VariantControl=V_i_6_8_w3_hti2
      link override alpha_i1/alpha_i_horizontal: VariantControl=V_i_6_8_w3_hti0
      link override alpha_i1/alpha_i_up: VariantControl=V_i_6_8_w3_hti1
      link override alpha_i2/alpha_i_down: VariantControl=V_i_6_8_w3_hti2
      link override alpha_i2/alpha_i_horizontal: VariantControl=V_i_6_8_w3_hti0
      link override alpha_i2/alpha_i_up: VariantControl=V_i_6_8_w3_hti1
  "[S1]" : Outport
  "[S2]" : Outport  Port=2

== system building_PHPP_v1/BUILDING/INTERSECTION_6_9/airexchange_1 ==
  AIB1 : Inport
  AIB2 : Inport  Port=2
  control : Inport  Port=3
  EMPTY : carnotUIBK/airexchange_intersection/EMPTY  VariantControl=(default)
  airexchange_empiric : carnotUIBK/airexchange_intersection/airexchange_empiric  VariantControl=V_i_6_9_inf1_m0
  airexchange_powerlaw : carnotUIBK/airexchange_intersection/airexchange_powerlaw  VariantControl=V_i_6_9_inf1_m1
  "[S1]" : Outport
  "[S2]" : Outport  Port=2
